simulink model "gm_rgb_gauss_sobel_64bit_full"  (R2022a)
settings: Solver=VariableStepAuto  StartTime=0.0  StopTime=10.0  RelTol=1e-3
undefined symbols (not defined in the file or in its folder): blueMax, blueMin, gray, greenMax, greenMin, redMax, redMin
libraries: hdlsllib x62, visionhdlio x6, visionsources x2
(part 3 of 3)

== system gm_rgb_gauss_sobel_64bit_full/Subsystem/conv_core_gauss/Subsystem1/slicer R operation3/Line buffer1 ==
  in0 : Inport  OutDataTypeStr=fixdt(0,8,0,'DataTypeOverride', 'Off')  SampleTime=2.77039007092199e-06
  <valid> : EnablePort  OutDataTypeStr=boolean
  Line buffer1 : Delay  DelayLength=double(750)  InitialCondition=0
  out0 : Outport  OutDataTypeStr=uint8  SampleTime=2.77039007092199e-06  InitialOutput=0
  wires:
  Line buffer1/1 -> out0/1
  in0/1 -> Line buffer1/1

== system gm_rgb_gauss_sobel_64bit_full/Subsystem/conv_core_gauss/Subsystem1/slicer R operation4/Delay1 ==
  in0 : Inport  OutDataTypeStr=fixdt(0,8,0,'DataTypeOverride', 'Off')  SampleTime=2.77039007092199e-06
  <valid> : EnablePort  OutDataTypeStr=boolean
  Delay1 : Delay  DelayLength=double(1)  InitialCondition=0
  out0 : Outport  OutDataTypeStr=uint8  SampleTime=2.77039007092199e-06  InitialOutput=0
  wires:
  Delay1/1 -> out0/1
  in0/1 -> Delay1/1

== system gm_rgb_gauss_sobel_64bit_full/Subsystem/conv_core_gauss/Subsystem1/slicer R operation4/Delay2 ==
  in0 : Inport  OutDataTypeStr=fixdt(0,8,0,'DataTypeOverride', 'Off')  SampleTime=2.77039007092199e-06
  <valid> : EnablePort  OutDataTypeStr=boolean
  Delay2 : Delay  DelayLength=double(1)  InitialCondition=0
  out0 : Outport  OutDataTypeStr=uint8  SampleTime=2.77039007092199e-06  InitialOutput=0
  wires:
  Delay2/1 -> out0/1
  in0/1 -> Delay2/1

== system gm_rgb_gauss_sobel_64bit_full/Subsystem/conv_core_gauss/Subsystem1/slicer R operation4/Delay3 ==
  in0 : Inport  OutDataTypeStr=fixdt(0,8,0,'DataTypeOverride', 'Off')  SampleTime=2.77039007092199e-06
  <valid> : EnablePort  OutDataTypeStr=boolean
  Delay3 : Delay  DelayLength=double(1)  InitialCondition=0
  out0 : Outport  OutDataTypeStr=uint8  SampleTime=2.77039007092199e-06  InitialOutput=0
  wires:
  Delay3/1 -> out0/1
  in0/1 -> Delay3/1

== system gm_rgb_gauss_sobel_64bit_full/Subsystem/conv_core_gauss/Subsystem1/slicer R operation4/Delay4 ==
  in0 : Inport  OutDataTypeStr=fixdt(0,8,0,'DataTypeOverride', 'Off')  SampleTime=2.77039007092199e-06
  <valid> : EnablePort  OutDataTypeStr=boolean
  Delay4 : Delay  DelayLength=double(1)  InitialCondition=0
  out0 : Outport  OutDataTypeStr=uint8  SampleTime=2.77039007092199e-06  InitialOutput=0
  wires:
  Delay4/1 -> out0/1
  in0/1 -> Delay4/1

== system gm_rgb_gauss_sobel_64bit_full/Subsystem/conv_core_gauss/Subsystem1/slicer R operation4/Delay5 ==
  in0 : Inport  OutDataTypeStr=fixdt(0,8,0,'DataTypeOverride', 'Off')  SampleTime=2.77039007092199e-06
  <valid> : EnablePort  OutDataTypeStr=boolean
  Delay5 : Delay  DelayLength=double(1)  InitialCondition=0
  out0 : Outport  OutDataTypeStr=uint8  SampleTime=2.77039007092199e-06  InitialOutput=0
  wires:
  Delay5/1 -> out0/1
  in0/1 -> Delay5/1

== system gm_rgb_gauss_sobel_64bit_full/Subsystem/conv_core_gauss/Subsystem1/slicer R operation4/Delay6 ==
  in0 : Inport  OutDataTypeStr=fixdt(0,8,0,'DataTypeOverride', 'Off')  SampleTime=2.77039007092199e-06
  <valid> : EnablePort  OutDataTypeStr=boolean
  Delay6 : Delay  DelayLength=double(1)  InitialCondition=0
  out0 : Outport  OutDataTypeStr=uint8  SampleTime=2.77039007092199e-06  InitialOutput=0
  wires:
  Delay6/1 -> out0/1
  in0/1 -> Delay6/1

== system gm_rgb_gauss_sobel_64bit_full/Subsystem/conv_core_gauss/Subsystem1/slicer R operation4/Line buffer ==
  in0 : Inport  OutDataTypeStr=fixdt(0,8,0,'DataTypeOverride', 'Off')  SampleTime=2.77039007092199e-06
  <valid> : EnablePort  OutDataTypeStr=boolean
  Line buffer : Delay  DelayLength=double(750)  InitialCondition=0
  out0 : Outport  OutDataTypeStr=uint8  SampleTime=2.77039007092199e-06  InitialOutput=0
  wires:
  Line buffer/1 -> out0/1
  in0/1 -> Line buffer/1

== system gm_rgb_gauss_sobel_64bit_full/Subsystem/conv_core_gauss/Subsystem1/slicer R operation4/Line buffer1 ==
  in0 : Inport  OutDataTypeStr=fixdt(0,8,0,'DataTypeOverride', 'Off')  SampleTime=2.77039007092199e-06
  <valid> : EnablePort  OutDataTypeStr=boolean
  Line buffer1 : Delay  DelayLength=double(750)  InitialCondition=0
  out0 : Outport  OutDataTypeStr=uint8  SampleTime=2.77039007092199e-06  InitialOutput=0
  wires:
  Line buffer1/1 -> out0/1
  in0/1 -> Line buffer1/1

== system gm_rgb_gauss_sobel_64bit_full/Subsystem/conv_core_gauss/Subsystem1/slicer R operation5/Delay1 ==
  in0 : Inport  OutDataTypeStr=fixdt(0,8,0,'DataTypeOverride', 'Off')  SampleTime=2.77039007092199e-06
  <valid> : EnablePort  OutDataTypeStr=boolean
  Delay1 : Delay  DelayLength=double(1)  InitialCondition=0
  out0 : Outport  OutDataTypeStr=uint8  SampleTime=2.77039007092199e-06  InitialOutput=0
  wires:
  Delay1/1 -> out0/1
  in0/1 -> Delay1/1

== system gm_rgb_gauss_sobel_64bit_full/Subsystem/conv_core_gauss/Subsystem1/slicer R operation5/Delay2 ==
  in0 : Inport  OutDataTypeStr=fixdt(0,8,0,'DataTypeOverride', 'Off')  SampleTime=2.77039007092199e-06
  <valid> : EnablePort  OutDataTypeStr=boolean
  Delay2 : Delay  DelayLength=double(1)  InitialCondition=0
  out0 : Outport  OutDataTypeStr=uint8  SampleTime=2.77039007092199e-06  InitialOutput=0
  wires:
  Delay2/1 -> out0/1
  in0/1 -> Delay2/1

== system gm_rgb_gauss_sobel_64bit_full/Subsystem/conv_core_gauss/Subsystem1/slicer R operation5/Delay3 ==
  in0 : Inport  OutDataTypeStr=fixdt(0,8,0,'DataTypeOverride', 'Off')  SampleTime=2.77039007092199e-06
  <valid> : EnablePort  OutDataTypeStr=boolean
  Delay3 : Delay  DelayLength=double(1)  InitialCondition=0
  out0 : Outport  OutDataTypeStr=uint8  SampleTime=2.77039007092199e-06  InitialOutput=0
  wires:
  Delay3/1 -> out0/1
  in0/1 -> Delay3/1

== system gm_rgb_gauss_sobel_64bit_full/Subsystem/conv_core_gauss/Subsystem1/slicer R operation5/Delay4 ==
  in0 : Inport  OutDataTypeStr=fixdt(0,8,0,'DataTypeOverride', 'Off')  SampleTime=2.77039007092199e-06
  <valid> : EnablePort  OutDataTypeStr=boolean
  Delay4 : Delay  DelayLength=double(1)  InitialCondition=0
  out0 : Outport  OutDataTypeStr=uint8  SampleTime=2.77039007092199e-06  InitialOutput=0
  wires:
  Delay4/1 -> out0/1
  in0/1 -> Delay4/1

== system gm_rgb_gauss_sobel_64bit_full/Subsystem/conv_core_gauss/Subsystem1/slicer R operation5/Delay5 ==
  in0 : Inport  OutDataTypeStr=fixdt(0,8,0,'DataTypeOverride', 'Off')  SampleTime=2.77039007092199e-06
  <valid> : EnablePort  OutDataTypeStr=boolean
  Delay5 : Delay  DelayLength=double(1)  InitialCondition=0
  out0 : Outport  OutDataTypeStr=uint8  SampleTime=2.77039007092199e-06  InitialOutput=0
  wires:
  Delay5/1 -> out0/1
  in0/1 -> Delay5/1

== system gm_rgb_gauss_sobel_64bit_full/Subsystem/conv_core_gauss/Subsystem1/slicer R operation5/Delay6 ==
  in0 : Inport  OutDataTypeStr=fixdt(0,8,0,'DataTypeOverride', 'Off')  SampleTime=2.77039007092199e-06
  <valid> : EnablePort  OutDataTypeStr=boolean
  Delay6 : Delay  DelayLength=double(1)  InitialCondition=0
  out0 : Outport  OutDataTypeStr=uint8  SampleTime=2.77039007092199e-06  InitialOutput=0
  wires:
  Delay6/1 -> out0/1
  in0/1 -> Delay6/1

== system gm_rgb_gauss_sobel_64bit_full/Subsystem/conv_core_gauss/Subsystem1/slicer R operation5/Line buffer ==
  in0 : Inport  OutDataTypeStr=fixdt(0,8,0,'DataTypeOverride', 'Off')  SampleTime=2.77039007092199e-06
  <valid> : EnablePort  OutDataTypeStr=boolean
  Line buffer : Delay  DelayLength=double(750)  InitialCondition=0
  out0 : Outport  OutDataTypeStr=uint8  SampleTime=2.77039007092199e-06  InitialOutput=0
  wires:
  Line buffer/1 -> out0/1
  in0/1 -> Line buffer/1

== system gm_rgb_gauss_sobel_64bit_full/Subsystem/conv_core_gauss/Subsystem1/slicer R operation5/Line buffer1 ==
  in0 : Inport  OutDataTypeStr=fixdt(0,8,0,'DataTypeOverride', 'Off')  SampleTime=2.77039007092199e-06
  <valid> : EnablePort  OutDataTypeStr=boolean
  Line buffer1 : Delay  DelayLength=double(750)  InitialCondition=0
  out0 : Outport  OutDataTypeStr=uint8  SampleTime=2.77039007092199e-06  InitialOutput=0
  wires:
  Line buffer1/1 -> out0/1
  in0/1 -> Line buffer1/1

== system gm_rgb_gauss_sobel_64bit_full/Subsystem/conv_core_gauss/Subsystem1/slicer R operation6/Delay1 ==
  in0 : Inport  OutDataTypeStr=fixdt(0,8,0,'DataTypeOverride', 'Off')  SampleTime=2.77039007092199e-06
  <valid> : EnablePort  OutDataTypeStr=boolean
  Delay1 : Delay  DelayLength=double(1)  InitialCondition=0
  out0 : Outport  OutDataTypeStr=uint8  SampleTime=2.77039007092199e-06  InitialOutput=0
  wires:
  Delay1/1 -> out0/1
  in0/1 -> Delay1/1

== system gm_rgb_gauss_sobel_64bit_full/Subsystem/conv_core_gauss/Subsystem1/slicer R operation6/Delay2 ==
  in0 : Inport  OutDataTypeStr=fixdt(0,8,0,'DataTypeOverride', 'Off')  SampleTime=2.77039007092199e-06
  <valid> : EnablePort  OutDataTypeStr=boolean
  Delay2 : Delay  DelayLength=double(1)  InitialCondition=0
  out0 : Outport  OutDataTypeStr=uint8  SampleTime=2.77039007092199e-06  InitialOutput=0
  wires:
  Delay2/1 -> out0/1
  in0/1 -> Delay2/1

== system gm_rgb_gauss_sobel_64bit_full/Subsystem/conv_core_gauss/Subsystem1/slicer R operation6/Delay3 ==
  in0 : Inport  OutDataTypeStr=fixdt(0,8,0,'DataTypeOverride', 'Off')  SampleTime=2.77039007092199e-06
  <valid> : EnablePort  OutDataTypeStr=boolean
  Delay3 : Delay  DelayLength=double(1)  InitialCondition=0
  out0 : Outport  OutDataTypeStr=uint8  SampleTime=2.77039007092199e-06  InitialOutput=0
  wires:
  Delay3/1 -> out0/1
  in0/1 -> Delay3/1

== system gm_rgb_gauss_sobel_64bit_full/Subsystem/conv_core_gauss/Subsystem1/slicer R operation6/Delay4 ==
  in0 : Inport  OutDataTypeStr=fixdt(0,8,0,'DataTypeOverride', 'Off')  SampleTime=2.77039007092199e-06
  <valid> : EnablePort  OutDataTypeStr=boolean
  Delay4 : Delay  DelayLength=double(1)  InitialCondition=0
  out0 : Outport  OutDataTypeStr=uint8  SampleTime=2.77039007092199e-06  InitialOutput=0
  wires:
  Delay4/1 -> out0/1
  in0/1 -> Delay4/1

== system gm_rgb_gauss_sobel_64bit_full/Subsystem/conv_core_gauss/Subsystem1/slicer R operation6/Delay5 ==
  in0 : Inport  OutDataTypeStr=fixdt(0,8,0,'DataTypeOverride', 'Off')  SampleTime=2.77039007092199e-06
  <valid> : EnablePort  OutDataTypeStr=boolean
  Delay5 : Delay  DelayLength=double(1)  InitialCondition=0
  out0 : Outport  OutDataTypeStr=uint8  SampleTime=2.77039007092199e-06  InitialOutput=0
  wires:
  Delay5/1 -> out0/1
  in0/1 -> Delay5/1

== system gm_rgb_gauss_sobel_64bit_full/Subsystem/conv_core_gauss/Subsystem1/slicer R operation6/Delay6 ==
  in0 : Inport  OutDataTypeStr=fixdt(0,8,0,'DataTypeOverride', 'Off')  SampleTime=2.77039007092199e-06
  <valid> : EnablePort  OutDataTypeStr=boolean
  Delay6 : Delay  DelayLength=double(1)  InitialCondition=0
  out0 : Outport  OutDataTypeStr=uint8  SampleTime=2.77039007092199e-06  InitialOutput=0
  wires:
  Delay6/1 -> out0/1
  in0/1 -> Delay6/1

== system gm_rgb_gauss_sobel_64bit_full/Subsystem/conv_core_gauss/Subsystem1/slicer R operation6/Line buffer ==
  in0 : Inport  OutDataTypeStr=fixdt(0,8,0,'DataTypeOverride', 'Off')  SampleTime=2.77039007092199e-06
  <valid> : EnablePort  OutDataTypeStr=boolean
  Line buffer : Delay  DelayLength=double(750)  InitialCondition=0
  out0 : Outport  OutDataTypeStr=uint8  SampleTime=2.77039007092199e-06  InitialOutput=0
  wires:
  Line buffer/1 -> out0/1
  in0/1 -> Line buffer/1

== system gm_rgb_gauss_sobel_64bit_full/Subsystem/conv_core_gauss/Subsystem1/slicer R operation6/Line buffer1 ==
  in0 : Inport  OutDataTypeStr=fixdt(0,8,0,'DataTypeOverride', 'Off')  SampleTime=2.77039007092199e-06
  <valid> : EnablePort  OutDataTypeStr=boolean
  Line buffer1 : Delay  DelayLength=double(750)  InitialCondition=0
  out0 : Outport  OutDataTypeStr=uint8  SampleTime=2.77039007092199e-06  InitialOutput=0
  wires:
  Line buffer1/1 -> out0/1
  in0/1 -> Line buffer1/1

== system gm_rgb_gauss_sobel_64bit_full/Subsystem/conv_core_sobel1/Subsystem1/conv X/Delay1 ==
  in0 : Inport  OutDataTypeStr=fixdt(1,16,0,'DataTypeOverride', 'Off')  PortDimensions=[9]  SampleTime=2.77039007092199e-06
  <valid> : EnablePort  OutDataTypeStr=boolean
  Delay1 : Delay  DelayLength=double(1)  InitialCondition=0
  out0 : Outport  OutDataTypeStr=int16  PortDimensions=[9]  SampleTime=2.77039007092199e-06  InitialOutput=0
  wires:
  Delay1/1 -> out0/1
  in0/1 -> Delay1/1

== system gm_rgb_gauss_sobel_64bit_full/Subsystem/conv_core_sobel1/Subsystem1/conv X/Delay2 ==
  in0 : Inport  OutDataTypeStr=fixdt(1,16,0,'DataTypeOverride', 'Off')  PortDimensions=[9]  SampleTime=2.77039007092199e-06
  <valid> : EnablePort  OutDataTypeStr=boolean
  Delay2 : Delay  DelayLength=double(1)  InitialCondition=0
  out0 : Outport  OutDataTypeStr=int16  PortDimensions=[9]  SampleTime=2.77039007092199e-06  InitialOutput=0
  wires:
  Delay2/1 -> out0/1
  in0/1 -> Delay2/1

== system gm_rgb_gauss_sobel_64bit_full/Subsystem/conv_core_sobel1/Subsystem1/conv X/Delay3 ==
  in0 : Inport  OutDataTypeStr=fixdt(0,8,0,'DataTypeOverride', 'Off')  SampleTime=2.77039007092199e-06
  <valid> : EnablePort  OutDataTypeStr=boolean
  Delay3 : Delay  DelayLength=double(1)  InitialCondition=0
  out0 : Outport  OutDataTypeStr=uint8  SampleTime=2.77039007092199e-06  InitialOutput=0
  wires:
  Delay3/1 -> out0/1
  in0/1 -> Delay3/1

== system gm_rgb_gauss_sobel_64bit_full/Subsystem/conv_core_sobel1/Subsystem1/conv X/Delay4 ==
  in0 : Inport  OutDataTypeStr=fixdt(0,8,0,'DataTypeOverride', 'Off')  SampleTime=2.77039007092199e-06
  <valid> : EnablePort  OutDataTypeStr=boolean
  Delay4 : Delay  DelayLength=double(1)  InitialCondition=0
  out0 : Outport  OutDataTypeStr=uint8  SampleTime=2.77039007092199e-06  InitialOutput=0
  wires:
  Delay4/1 -> out0/1
  in0/1 -> Delay4/1

== system gm_rgb_gauss_sobel_64bit_full/Subsystem/conv_core_sobel1/Subsystem1/conv X1/Delay1 ==
  in0 : Inport  OutDataTypeStr=fixdt(1,16,0,'DataTypeOverride', 'Off')  PortDimensions=[9]  SampleTime=2.77039007092199e-06
  <valid> : EnablePort  OutDataTypeStr=boolean
  Delay1 : Delay  DelayLength=double(1)  InitialCondition=0
  out0 : Outport  OutDataTypeStr=int16  PortDimensions=[9]  SampleTime=2.77039007092199e-06  InitialOutput=0
  wires:
  Delay1/1 -> out0/1
  in0/1 -> Delay1/1

== system gm_rgb_gauss_sobel_64bit_full/Subsystem/conv_core_sobel1/Subsystem1/conv X1/Delay2 ==
  in0 : Inport  OutDataTypeStr=fixdt(1,16,0,'DataTypeOverride', 'Off')  PortDimensions=[9]  SampleTime=2.77039007092199e-06
  <valid> : EnablePort  OutDataTypeStr=boolean
  Delay2 : Delay  DelayLength=double(1)  InitialCondition=0
  out0 : Outport  OutDataTypeStr=int16  PortDimensions=[9]  SampleTime=2.77039007092199e-06  InitialOutput=0
  wires:
  Delay2/1 -> out0/1
  in0/1 -> Delay2/1

== system gm_rgb_gauss_sobel_64bit_full/Subsystem/conv_core_sobel1/Subsystem1/conv X1/Delay3 ==
  in0 : Inport  OutDataTypeStr=fixdt(0,8,0,'DataTypeOverride', 'Off')  SampleTime=2.77039007092199e-06
  <valid> : EnablePort  OutDataTypeStr=boolean
  Delay3 : Delay  DelayLength=double(1)  InitialCondition=0
  out0 : Outport  OutDataTypeStr=uint8  SampleTime=2.77039007092199e-06  InitialOutput=0
  wires:
  Delay3/1 -> out0/1
  in0/1 -> Delay3/1

== system gm_rgb_gauss_sobel_64bit_full/Subsystem/conv_core_sobel1/Subsystem1/conv X1/Delay4 ==
  in0 : Inport  OutDataTypeStr=fixdt(0,8,0,'DataTypeOverride', 'Off')  SampleTime=2.77039007092199e-06
  <valid> : EnablePort  OutDataTypeStr=boolean
  Delay4 : Delay  DelayLength=double(1)  InitialCondition=0
  out0 : Outport  OutDataTypeStr=uint8  SampleTime=2.77039007092199e-06  InitialOutput=0
  wires:
  Delay4/1 -> out0/1
  in0/1 -> Delay4/1

== system gm_rgb_gauss_sobel_64bit_full/Subsystem/conv_core_sobel1/Subsystem1/conv Y/Delay1 ==
  in0 : Inport  OutDataTypeStr=fixdt(1,16,0,'DataTypeOverride', 'Off')  PortDimensions=[9]  SampleTime=2.77039007092199e-06
  <valid> : EnablePort  OutDataTypeStr=boolean
  Delay1 : Delay  DelayLength=double(1)  InitialCondition=0
  out0 : Outport  OutDataTypeStr=int16  PortDimensions=[9]  SampleTime=2.77039007092199e-06  InitialOutput=0
  wires:
  Delay1/1 -> out0/1
  in0/1 -> Delay1/1

== system gm_rgb_gauss_sobel_64bit_full/Subsystem/conv_core_sobel1/Subsystem1/conv Y/Delay2 ==
  in0 : Inport  OutDataTypeStr=fixdt(1,16,0,'DataTypeOverride', 'Off')  PortDimensions=[9]  SampleTime=2.77039007092199e-06
  <valid> : EnablePort  OutDataTypeStr=boolean
  Delay2 : Delay  DelayLength=double(1)  InitialCondition=0
  out0 : Outport  OutDataTypeStr=int16  PortDimensions=[9]  SampleTime=2.77039007092199e-06  InitialOutput=0
  wires:
  Delay2/1 -> out0/1
  in0/1 -> Delay2/1

== system gm_rgb_gauss_sobel_64bit_full/Subsystem/conv_core_sobel1/Subsystem1/conv Y/Delay4 ==
  in0 : Inport  OutDataTypeStr=fixdt(0,8,0,'DataTypeOverride', 'Off')  SampleTime=2.77039007092199e-06
  <valid> : EnablePort  OutDataTypeStr=boolean
  Delay4 : Delay  DelayLength=double(1)  InitialCondition=0
  out0 : Outport  OutDataTypeStr=uint8  SampleTime=2.77039007092199e-06  InitialOutput=0
  wires:
  Delay4/1 -> out0/1
  in0/1 -> Delay4/1

== system gm_rgb_gauss_sobel_64bit_full/Subsystem/conv_core_sobel1/Subsystem1/conv Y/Delay5 ==
  in0 : Inport  OutDataTypeStr=fixdt(0,8,0,'DataTypeOverride', 'Off')  SampleTime=2.77039007092199e-06
  <valid> : EnablePort  OutDataTypeStr=boolean
  Delay5 : Delay  DelayLength=double(1)  InitialCondition=0
  out0 : Outport  OutDataTypeStr=uint8  SampleTime=2.77039007092199e-06  InitialOutput=0
  wires:
  Delay5/1 -> out0/1
  in0/1 -> Delay5/1

== system gm_rgb_gauss_sobel_64bit_full/Subsystem/conv_core_sobel1/Subsystem1/conv Y1/Delay1 ==
  in0 : Inport  OutDataTypeStr=fixdt(1,16,0,'DataTypeOverride', 'Off')  PortDimensions=[9]  SampleTime=2.77039007092199e-06
  <valid> : EnablePort  OutDataTypeStr=boolean
  Delay1 : Delay  DelayLength=double(1)  InitialCondition=0
  out0 : Outport  OutDataTypeStr=int16  PortDimensions=[9]  SampleTime=2.77039007092199e-06  InitialOutput=0
  wires:
  Delay1/1 -> out0/1
  in0/1 -> Delay1/1

== system gm_rgb_gauss_sobel_64bit_full/Subsystem/conv_core_sobel1/Subsystem1/conv Y1/Delay2 ==
  in0 : Inport  OutDataTypeStr=fixdt(1,16,0,'DataTypeOverride', 'Off')  PortDimensions=[9]  SampleTime=2.77039007092199e-06
  <valid> : EnablePort  OutDataTypeStr=boolean
  Delay2 : Delay  DelayLength=double(1)  InitialCondition=0
  out0 : Outport  OutDataTypeStr=int16  PortDimensions=[9]  SampleTime=2.77039007092199e-06  InitialOutput=0
  wires:
  Delay2/1 -> out0/1
  in0/1 -> Delay2/1

== system gm_rgb_gauss_sobel_64bit_full/Subsystem/conv_core_sobel1/Subsystem1/conv Y1/Delay4 ==
  in0 : Inport  OutDataTypeStr=fixdt(0,8,0,'DataTypeOverride', 'Off')  SampleTime=2.77039007092199e-06
  <valid> : EnablePort  OutDataTypeStr=boolean
  Delay4 : Delay  DelayLength=double(1)  InitialCondition=0
  out0 : Outport  OutDataTypeStr=uint8  SampleTime=2.77039007092199e-06  InitialOutput=0
  wires:
  Delay4/1 -> out0/1
  in0/1 -> Delay4/1

== system gm_rgb_gauss_sobel_64bit_full/Subsystem/conv_core_sobel1/Subsystem1/conv Y1/Delay5 ==
  in0 : Inport  OutDataTypeStr=fixdt(0,8,0,'DataTypeOverride', 'Off')  SampleTime=2.77039007092199e-06
  <valid> : EnablePort  OutDataTypeStr=boolean
  Delay5 : Delay  DelayLength=double(1)  InitialCondition=0
  out0 : Outport  OutDataTypeStr=uint8  SampleTime=2.77039007092199e-06  InitialOutput=0
  wires:
  Delay5/1 -> out0/1
  in0/1 -> Delay5/1

== system gm_rgb_gauss_sobel_64bit_full/Subsystem/conv_core_sobel1/Subsystem1/slicer L operation1/Delay1 ==
  in0 : Inport  OutDataTypeStr=fixdt(0,8,0,'DataTypeOverride', 'Off')  SampleTime=2.77039007092199e-06
  <valid> : EnablePort  OutDataTypeStr=boolean
  Delay1 : Delay  DelayLength=double(1)  InitialCondition=0
  out0 : Outport  OutDataTypeStr=uint8  SampleTime=2.77039007092199e-06  InitialOutput=0
  wires:
  Delay1/1 -> out0/1
  in0/1 -> Delay1/1

== system gm_rgb_gauss_sobel_64bit_full/Subsystem/conv_core_sobel1/Subsystem1/slicer L operation1/Delay2 ==
  in0 : Inport  OutDataTypeStr=fixdt(0,8,0,'DataTypeOverride', 'Off')  SampleTime=2.77039007092199e-06
  <valid> : EnablePort  OutDataTypeStr=boolean
  Delay2 : Delay  DelayLength=double(1)  InitialCondition=0
  out0 : Outport  OutDataTypeStr=uint8  SampleTime=2.77039007092199e-06  InitialOutput=0
  wires:
  Delay2/1 -> out0/1
  in0/1 -> Delay2/1

== system gm_rgb_gauss_sobel_64bit_full/Subsystem/conv_core_sobel1/Subsystem1/slicer L operation1/Delay3 ==
  in0 : Inport  OutDataTypeStr=fixdt(0,8,0,'DataTypeOverride', 'Off')  SampleTime=2.77039007092199e-06
  <valid> : EnablePort  OutDataTypeStr=boolean
  Delay3 : Delay  DelayLength=double(1)  InitialCondition=0
  out0 : Outport  OutDataTypeStr=uint8  SampleTime=2.77039007092199e-06  InitialOutput=0
  wires:
  Delay3/1 -> out0/1
  in0/1 -> Delay3/1

== system gm_rgb_gauss_sobel_64bit_full/Subsystem/conv_core_sobel1/Subsystem1/slicer L operation1/Delay4 ==
  in0 : Inport  OutDataTypeStr=fixdt(0,8,0,'DataTypeOverride', 'Off')  SampleTime=2.77039007092199e-06
  <valid> : EnablePort  OutDataTypeStr=boolean
  Delay4 : Delay  DelayLength=double(1)  InitialCondition=0
  out0 : Outport  OutDataTypeStr=uint8  SampleTime=2.77039007092199e-06  InitialOutput=0
  wires:
  Delay4/1 -> out0/1
  in0/1 -> Delay4/1

== system gm_rgb_gauss_sobel_64bit_full/Subsystem/conv_core_sobel1/Subsystem1/slicer L operation1/Delay5 ==
  in0 : Inport  OutDataTypeStr=fixdt(0,8,0,'DataTypeOverride', 'Off')  SampleTime=2.77039007092199e-06
  <valid> : EnablePort  OutDataTypeStr=boolean
  Delay5 : Delay  DelayLength=double(1)  InitialCondition=0
  out0 : Outport  OutDataTypeStr=uint8  SampleTime=2.77039007092199e-06  InitialOutput=0
  wires:
  Delay5/1 -> out0/1
  in0/1 -> Delay5/1

== system gm_rgb_gauss_sobel_64bit_full/Subsystem/conv_core_sobel1/Subsystem1/slicer L operation1/Delay6 ==
  in0 : Inport  OutDataTypeStr=fixdt(0,8,0,'DataTypeOverride', 'Off')  SampleTime=2.77039007092199e-06
  <valid> : EnablePort  OutDataTypeStr=boolean
  Delay6 : Delay  DelayLength=double(1)  InitialCondition=0
  out0 : Outport  OutDataTypeStr=uint8  SampleTime=2.77039007092199e-06  InitialOutput=0
  wires:
  Delay6/1 -> out0/1
  in0/1 -> Delay6/1

== system gm_rgb_gauss_sobel_64bit_full/Subsystem/conv_core_sobel1/Subsystem1/slicer L operation1/Line buffer ==
  in0 : Inport  OutDataTypeStr=fixdt(0,8,0,'DataTypeOverride', 'Off')  SampleTime=2.77039007092199e-06
  <valid> : EnablePort  OutDataTypeStr=boolean
  Line buffer : Delay  DelayLength=double(750)  InitialCondition=0
  out0 : Outport  OutDataTypeStr=uint8  SampleTime=2.77039007092199e-06  InitialOutput=0
  wires:
  Line buffer/1 -> out0/1
  in0/1 -> Line buffer/1

== system gm_rgb_gauss_sobel_64bit_full/Subsystem/conv_core_sobel1/Subsystem1/slicer L operation1/Line buffer1 ==
  in0 : Inport  OutDataTypeStr=fixdt(0,8,0,'DataTypeOverride', 'Off')  SampleTime=2.77039007092199e-06
  <valid> : EnablePort  OutDataTypeStr=boolean
  Line buffer1 : Delay  DelayLength=double(750)  InitialCondition=0
  out0 : Outport  OutDataTypeStr=uint8  SampleTime=2.77039007092199e-06  InitialOutput=0
  wires:
  Line buffer1/1 -> out0/1
  in0/1 -> Line buffer1/1

== system gm_rgb_gauss_sobel_64bit_full/Subsystem/conv_core_sobel1/Subsystem1/slicer R operation/Delay1 ==
  in0 : Inport  OutDataTypeStr=fixdt(0,8,0,'DataTypeOverride', 'Off')  SampleTime=2.77039007092199e-06
  <valid> : EnablePort  OutDataTypeStr=boolean
  Delay1 : Delay  DelayLength=double(1)  InitialCondition=0
  out0 : Outport  OutDataTypeStr=uint8  SampleTime=2.77039007092199e-06  InitialOutput=0
  wires:
  Delay1/1 -> out0/1
  in0/1 -> Delay1/1

== system gm_rgb_gauss_sobel_64bit_full/Subsystem/conv_core_sobel1/Subsystem1/slicer R operation/Delay2 ==
  in0 : Inport  OutDataTypeStr=fixdt(0,8,0,'DataTypeOverride', 'Off')  SampleTime=2.77039007092199e-06
  <valid> : EnablePort  OutDataTypeStr=boolean
  Delay2 : Delay  DelayLength=double(1)  InitialCondition=0
  out0 : Outport  OutDataTypeStr=uint8  SampleTime=2.77039007092199e-06  InitialOutput=0
  wires:
  Delay2/1 -> out0/1
  in0/1 -> Delay2/1

== system gm_rgb_gauss_sobel_64bit_full/Subsystem/conv_core_sobel1/Subsystem1/slicer R operation/Delay3 ==
  in0 : Inport  OutDataTypeStr=fixdt(0,8,0,'DataTypeOverride', 'Off')  SampleTime=2.77039007092199e-06
  <valid> : EnablePort  OutDataTypeStr=boolean
  Delay3 : Delay  DelayLength=double(1)  InitialCondition=0
  out0 : Outport  OutDataTypeStr=uint8  SampleTime=2.77039007092199e-06  InitialOutput=0
  wires:
  Delay3/1 -> out0/1
  in0/1 -> Delay3/1

== system gm_rgb_gauss_sobel_64bit_full/Subsystem/conv_core_sobel1/Subsystem1/slicer R operation/Delay4 ==
  in0 : Inport  OutDataTypeStr=fixdt(0,8,0,'DataTypeOverride', 'Off')  SampleTime=2.77039007092199e-06
  <valid> : EnablePort  OutDataTypeStr=boolean
  Delay4 : Delay  DelayLength=double(1)  InitialCondition=0
  out0 : Outport  OutDataTypeStr=uint8  SampleTime=2.77039007092199e-06  InitialOutput=0
  wires:
  Delay4/1 -> out0/1
  in0/1 -> Delay4/1

== system gm_rgb_gauss_sobel_64bit_full/Subsystem/conv_core_sobel1/Subsystem1/slicer R operation/Delay5 ==
  in0 : Inport  OutDataTypeStr=fixdt(0,8,0,'DataTypeOverride', 'Off')  SampleTime=2.77039007092199e-06
  <valid> : EnablePort  OutDataTypeStr=boolean
  Delay5 : Delay  DelayLength=double(1)  InitialCondition=0
  out0 : Outport  OutDataTypeStr=uint8  SampleTime=2.77039007092199e-06  InitialOutput=0
  wires:
  Delay5/1 -> out0/1
  in0/1 -> Delay5/1

== system gm_rgb_gauss_sobel_64bit_full/Subsystem/conv_core_sobel1/Subsystem1/slicer R operation/Delay6 ==
  in0 : Inport  OutDataTypeStr=fixdt(0,8,0,'DataTypeOverride', 'Off')  SampleTime=2.77039007092199e-06
  <valid> : EnablePort  OutDataTypeStr=boolean
  Delay6 : Delay  DelayLength=double(1)  InitialCondition=0
  out0 : Outport  OutDataTypeStr=uint8  SampleTime=2.77039007092199e-06  InitialOutput=0
  wires:
  Delay6/1 -> out0/1
  in0/1 -> Delay6/1

== system gm_rgb_gauss_sobel_64bit_full/Subsystem/conv_core_sobel1/Subsystem1/slicer R operation/Line buffer ==
  in0 : Inport  OutDataTypeStr=fixdt(0,8,0,'DataTypeOverride', 'Off')  SampleTime=2.77039007092199e-06
  <valid> : EnablePort  OutDataTypeStr=boolean
  Line buffer : Delay  DelayLength=double(750)  InitialCondition=0
  out0 : Outport  OutDataTypeStr=uint8  SampleTime=2.77039007092199e-06  InitialOutput=0
  wires:
  Line buffer/1 -> out0/1
  in0/1 -> Line buffer/1

== system gm_rgb_gauss_sobel_64bit_full/Subsystem/conv_core_sobel1/Subsystem1/slicer R operation/Line buffer1 ==
  in0 : Inport  OutDataTypeStr=fixdt(0,8,0,'DataTypeOverride', 'Off')  SampleTime=2.77039007092199e-06
  <valid> : EnablePort  OutDataTypeStr=boolean
  Line buffer1 : Delay  DelayLength=double(750)  InitialCondition=0
  out0 : Outport  OutDataTypeStr=uint8  SampleTime=2.77039007092199e-06  InitialOutput=0
  wires:
  Line buffer1/1 -> out0/1
  in0/1 -> Line buffer1/1
